simulink model "sixdof"  (R2022b)
settings: Solver=VariableStepAuto  StartTime=0.0  StopTime=10  RelTol=1e-3
undefined symbols (not defined in the file or in its folder): sigbuilder_block
libraries: matrix_library x1, shared6dof x1
settings Model: Creator=Freddie  LastModifiedBy=Freddie

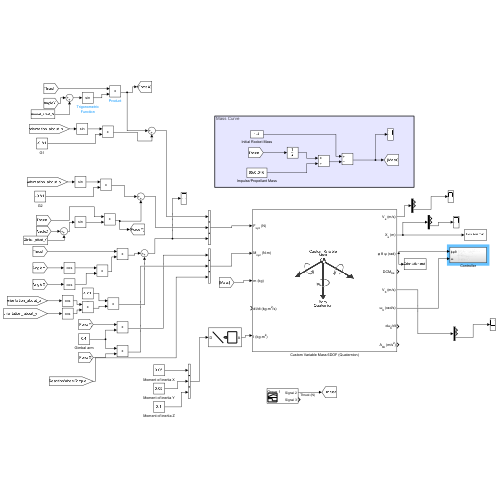
[thumbnail: Simulink's stored preview of the top-level diagram]
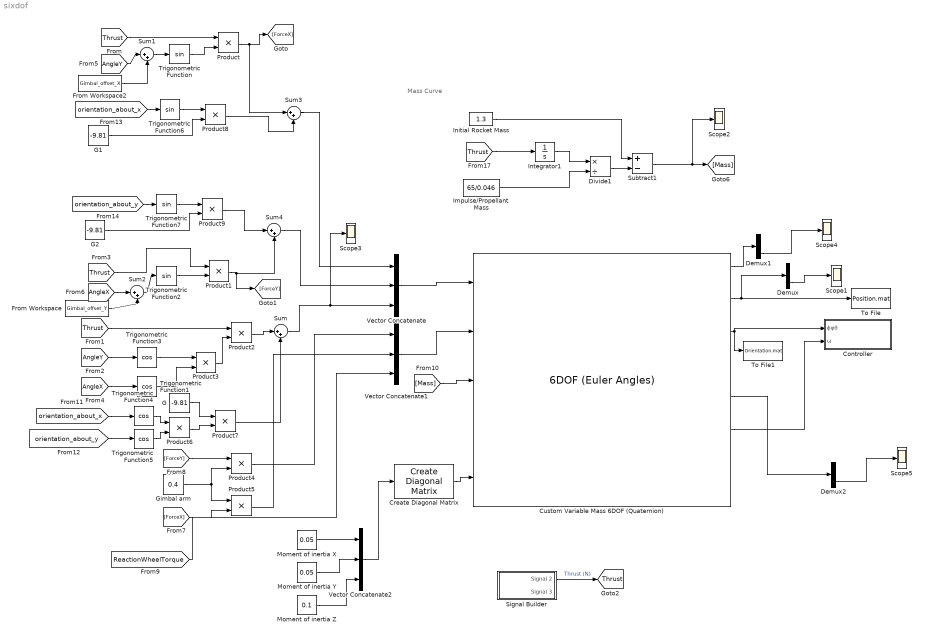
== system sixdof ==
  note: Mass Curve
  Controller : Subsystem
  Create Diagonal Matrix : matrix_library/Create Diagonal Matrix
      settings: LibrarySourceBlock=|
      | simulink/Matrix
      | Operations/Create Diagonal
      | Matrix
  Custom Variable Mass 6DOF (Quaternion) : shared6dof/6DOF (Euler Angles)  units=Metric (MKS)  mtype=Custom Variable  rep=Quaternion  xme_0=[0 0 0]  Vm_0=[0 0 0]  eul_0="[0 0 0  ]"  pm_0=[0 0 0]  mass_0=1.0  mass_e=0.5  mass_f=2.0  inertia=eye(3)  inertia_e=eye(3)  inertia_f=2*eye(3)  k_quat=1.0  vre_flag=off  abi_flag=off  aMode=0  xme_statename=''  Vm_statename=''  eul_statename=''  quat_statename=''  pm_statename=''  mass_statename=''
      settings: LibrarySourceBlock=aerolib6dof2/Custom Variable Mass 6DOF (Quaternion)
  Demux : Demux  Outputs=3
  Demux1 : Demux  Outputs=3
  Demux2 : Demux  Outputs=3
  Divide1 : Product  Inputs=*/
  From Workspace : FromWorkspace  VariableName=Gimbal_offset_Y  OutputAfterFinalValue=Holding final value
  From Workspace2 : FromWorkspace  VariableName=Gimbal_offset_X  OutputAfterFinalValue=Holding final value
  G : Constant  Value=-9.81
  G1 : Constant  Value=-9.81
  G2 : Constant  Value=-9.81
  Gimbal arm : Constant  Value=0.4
  Impulse/Propellant Mass : Constant  Value=65/0.046
  Initial Rocket Mass : Constant  Value=1.3
  Integrator1 : Integrator
  Moment of inertia X : Constant  Value=0.05
  Moment of inertia Y : Constant  Value=0.05
  Moment of inertia Z : Constant  Value=0.1
  Product{,1..9} (10 alike) : Product
  Scope{1..5} (5 alike) : Scope
  Signal Builder : Subsystem  Tag=STV Subsys  LoadFcn=sigbuilder_block('load');  StartFcn=sigbuilder_block('start');  StopFcn=sigbuilder_block('stop');  ClipboardFcn=sigbuilder_block('clipboard');  mask(Sigbuilder block){tuvar=[0:10]}
      mask help: Simulink:masks:SigbuilderBlock_MD
      mask init:
      | if ~strcmp(get_param(bdroot(gcbh),'SimulationStatus'),'stopped') tuvar = sigbuilder_block('maskInit'); end
      settings: CopyFcn=sigbuilder_block('copy');  DeleteFcn=sigbuilder_block('delete');  ModelCloseFcn=sigbuilder_block('modelClose');  PreSaveFcn=sigbuilder_block('preSave');  PauseFcn=sigbuilder_block('pause');  ContinueFcn=sigbuilder_block('continue');  NameChangeFcn=sigbuilder_block('namechange');  OpenFcn=sigbuilder_block('open',[437.6 199.2 550.4 400 ]);  CloseFcn=sigbuilder_block('close');
      mask Display: plot(0, 0, 100, 100,[2, 2, 32, 32, 2], [68, 8, 8, 68, 68],[32, 2], [38, 38], [32, 19, 2],[53, 60, 44], [32, 17, 17, 2],[16, 16, 31, 31]);txt = getActiveGroup(gcbh);text(2, 100, txt,'verticalAlignment', 'top');
  Subtract1 : Sum  Inputs=+-
  Sum{,1..4} (5 alike) : Sum  Inputs=|++
  To File : ToFile  Filename=Position.mat  MatrixName=Position  SampleTime=0.05
  To File1 : ToFile  Filename=Orientation.mat  MatrixName=Orientation  SampleTime=0.05
  Trigonometric Function{,2,6..7} (4 alike) : Trigonometry
  Trigonometric Function{1,3..5} (4 alike) : Trigonometry  Operator=cos
  Vector Concatenate : Concatenate  NumInputs=3
  Vector Concatenate1 : Concatenate  NumInputs=3
  Vector Concatenate2 : Concatenate  NumInputs=3
  tag scope: Thrust=global
  wires:
  [Thrust] -> Product/1
  Trigonometric Function/1 -> Product/2
  [Thrust] -> Product1/1
  Trigonometric Function2/1 -> Product1/2
  Trigonometric Function3/1 -> Product3/1
  Trigonometric Function1/1 -> Product3/2
  [Thrust] -> Product2/1
  Product3/1 -> Product2/2
  Product/1 -> Sum3/1, [ForceX]
  Product1/1 -> Sum4/2, [ForceY]
  [AngleY] -> Trigonometric Function3/1
  [AngleX] -> Trigonometric Function1/1
  Vector Concatenate/1 -> Custom Variable Mass 6DOF (Quaternion)/1
  Vector Concatenate1/1 -> Custom Variable Mass 6DOF (Quaternion)/2
  [ForceY] -> Product4/1
  [ForceX] -> Product5/2
  Gimbal arm/1 -> Product4/2, Product5/1
  [ReactionWheelTorque] -> Vector Concatenate1/3
  Signal Builder/1(Signal 2) -> [Thrust]  "Thrust (N)"
  Product2/1 -> Sum/1
  [Thrust] -> Integrator1/1
  Integrator1/1 -> Divide1/1
  Subtract1/1 -> Scope2/1, [Mass]
  Initial Rocket Mass/1 -> Subtract1/1
  Divide1/1 -> Subtract1/2
  Impulse/Propellant Mass/1 -> Divide1/2
  [Mass] -> Custom Variable Mass 6DOF (Quaternion)/3
  Create Diagonal Matrix/1 -> Custom Variable Mass 6DOF (Quaternion)/5
  Vector Concatenate2/1 -> Create Diagonal Matrix/1
  Moment of inertia Z/1 -> Vector Concatenate2/3
  Sum/1 -> Vector Concatenate/3, Scope3/1
  [AngleY] -> Sum1/1
  Sum1/1 -> Trigonometric Function/1
  [AngleX] -> Sum2/1
  Sum2/1 -> Trigonometric Function2/1
  From Workspace/1 -> Sum2/2
  From Workspace2/1 -> Sum1/2
  Custom Variable Mass 6DOF (Quaternion)/2 -> Demux/1, To File/1
  Custom Variable Mass 6DOF (Quaternion)/3 -> Controller/1(ϕφθ), To File1/1
  Custom Variable Mass 6DOF (Quaternion)/6 -> Controller/2(ω)
  Moment of inertia X/1 -> Vector Concatenate2/1
  Moment of inertia Y/1 -> Vector Concatenate2/2
  Product4/1 -> Vector Concatenate1/1
  Product5/1 -> Vector Concatenate1/2
  Demux/3 -> Scope1/1
  Custom Variable Mass 6DOF (Quaternion)/1 -> Demux1/1
  Demux1/3 -> Scope4/1
  Demux2/3 -> Scope5/1
  [orientation_about_x] -> Trigonometric Function4/1
  [orientation_about_y] -> Trigonometric Function5/1
  Trigonometric Function4/1 -> Product6/1
  Trigonometric Function5/1 -> Product6/2
  Product6/1 -> Product7/2
  G/1 -> Product7/1
  Product7/1 -> Sum/2
  [orientation_about_x] -> Trigonometric Function6/1
  Trigonometric Function6/1 -> Product8/1
  G1/1 -> Product8/2
  Product8/1 -> Sum3/2
  Sum3/1 -> Vector Concatenate/1
  [orientation_about_y] -> Trigonometric Function7/1
  Trigonometric Function7/1 -> Product9/1
  G2/1 -> Product9/2
  Product9/1 -> Sum4/1
  Sum4/1 -> Vector Concatenate/2
  Custom Variable Mass 6DOF (Quaternion)/5 -> Demux2/1

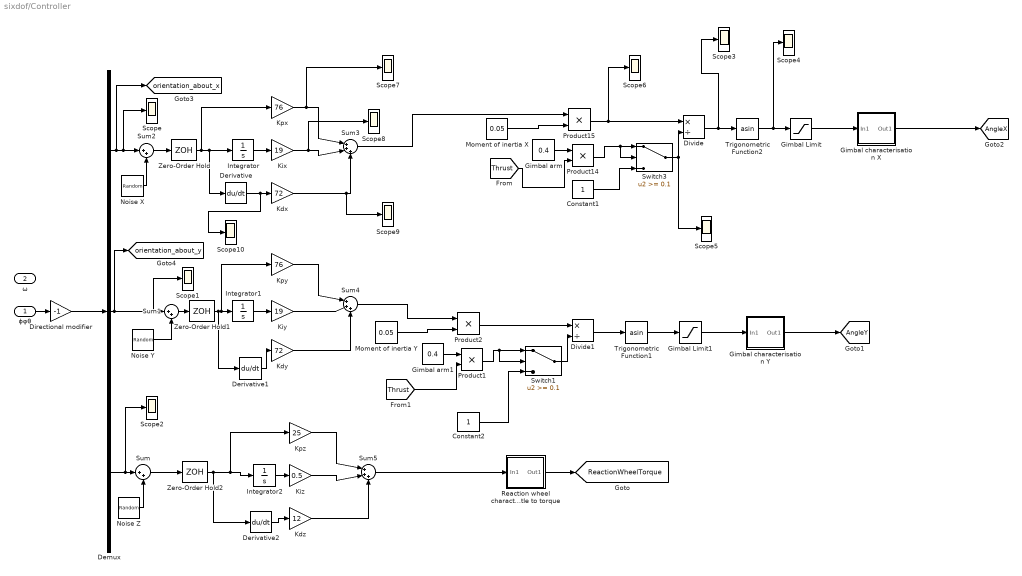
== system sixdof/Controller ==
  ϕφθ : Inport
  ω : Inport  Port=2
  Constant1 : Constant
  Constant2 : Constant
  Demux : Demux  Outputs=3
  Derivative : Derivative
  Derivative1 : Derivative
  Derivative2 : Derivative
  Directional modifier : Gain  Gain=-1
  Divide : Product  Inputs=*/
  Divide1 : Product  Inputs=*/
  Gimbal Limit : Saturate  UpperLimit=0.139626  LowerLimit=-0.139626
  Gimbal Limit1 : Saturate  UpperLimit=0.139626  LowerLimit=-0.139626
  Gimbal arm : Constant  Value=0.4
  Gimbal arm1 : Constant  Value=0.4
  Gimbal characterisation X : Subsystem
  Gimbal characterisation Y : Subsystem
  Integrator : Integrator
  Integrator1 : Integrator
  Integrator2 : Integrator
  Kdx : Gain  Gain=72
  Kdy : Gain  Gain=72
  Kdz : Gain  Gain=12
  Kix : Gain  Gain=19
  Kiy : Gain  Gain=19
  Kiz : Gain  Gain=0.5
  Kpx : Gain  Gain=76
  Kpy : Gain  Gain=76
  Kpz : Gain  Gain=25
  Moment of inertia X : Constant  Value=0.05
  Moment of inertia Y : Constant  Value=0.05
  Noise X : RandomNumber  Variance=0  SampleTime=0.1
  Noise Y : RandomNumber  Variance=0  SampleTime=0.1
  Noise Z : RandomNumber  Variance=0  Seed=2  SampleTime=0.1
  Product{1..2,14..15} (4 alike) : Product
  Reaction wheel characterization throttle to torque : Subsystem
  Scope{,1..10} (11 alike) : Scope
  Sum : Sum  Inputs=|++
  Sum1 : Sum  Inputs=|++
  Sum2 : Sum  Inputs=|++
  Sum3 : Sum  Inputs=|+++
  Sum4 : Sum  Inputs=|+++
  Sum5 : Sum  Inputs=|+++
  Switch1 : Switch  Threshold=0.1  SaturateOnIntegerOverflow=off  InputSameDT=off
  Switch3 : Switch  Threshold=0.1  SaturateOnIntegerOverflow=off  InputSameDT=off
  Trigonometric Function1 : Trigonometry  Operator=asin  OutputSignalType=real
  Trigonometric Function2 : Trigonometry  Operator=asin  OutputSignalType=real
  Zero-Order Hold : ZeroOrderHold  SampleTime=0.01
  Zero-Order Hold1 : ZeroOrderHold  SampleTime=0.01
  Zero-Order Hold2 : ZeroOrderHold  SampleTime=0.01
  tag scope: AngleX=global, AngleY=global, ReactionWheelTorque=global, orientation_about_x=global, orientation_about_y=global
  wires:
  Demux/3 -> Scope2/1, Sum/1
  Demux/1 -> [orientation_about_x], Scope/1, Sum2/1
  Demux/2 -> Scope1/1, Sum1/1, [orientation_about_y]
  Noise X/1 -> Sum2/2
  Noise Y/1 -> Sum1/2
  Noise Z/1 -> Sum/2
  Divide/1 -> Scope3/1, Trigonometric Function2/1
  Gimbal Limit/1 -> Gimbal characterisation X/1(In1)
  Product15/1 -> Scope6/1, Divide/1
  Trigonometric Function2/1 -> Scope4/1, Gimbal Limit/1
  Moment of inertia X/1 -> Product15/2
  Constant1/1 -> Switch3/3
  Gimbal arm/1 -> Product14/1
  Product14/1 -> Switch3/2, Switch3/1
  Switch3/1 -> Divide/2, Scope5/1
  Gimbal arm1/1 -> Product1/1
  Divide1/1 -> Trigonometric Function1/1
  Product2/1 -> Divide1/1
  Gimbal Limit1/1 -> Gimbal characterisation Y/1(In1)
  Trigonometric Function1/1 -> Gimbal Limit1/1
  Switch1/1 -> Divide1/2
  Constant2/1 -> Switch1/3
  Moment of inertia Y/1 -> Product2/2
  Reaction wheel characterization throttle to torque/1(Out1) -> [ReactionWheelTorque]
  Gimbal characterisation Y/1(Out1) -> [AngleY]
  Gimbal characterisation X/1(Out1) -> [AngleX]
  [Thrust] -> Product14/2
  [Thrust] -> Product1/2
  Product1/1 -> Switch1/2, Switch1/1
  Kpx/1 -> Scope7/1, Sum3/1
  Kix/1 -> Scope8/1, Sum3/2
  Kdx/1 -> Scope9/1, Sum3/3
  Kiy/1 -> Sum4/2
  Kpy/1 -> Sum4/1
  Kdy/1 -> Sum4/3
  Kiz/1 -> Sum5/2
  Kdz/1 -> Sum5/3
  Kpz/1 -> Sum5/1
  Sum5/1 -> Reaction wheel characterization throttle to torque/1(In1)
  Sum4/1 -> Product2/1
  Sum3/1 -> Product15/1
  Sum2/1 -> Zero-Order Hold/1
  Zero-Order Hold/1 -> Kpx/1, Derivative/1, Integrator/1
  Sum1/1 -> Zero-Order Hold1/1
  Zero-Order Hold1/1 -> Derivative1/1, Kpy/1, Integrator1/1
  Sum/1 -> Zero-Order Hold2/1
  Zero-Order Hold2/1 -> Derivative2/1, Kpz/1, Integrator2/1
  Integrator/1 -> Kix/1
  Integrator1/1 -> Kiy/1
  Integrator2/1 -> Kiz/1
  ϕφθ/1 -> Directional modifier/1
  Directional modifier/1 -> Demux/1
  Derivative1/1 -> Kdy/1
  Derivative2/1 -> Kdz/1
  Derivative/1 -> Scope10/1, Kdx/1

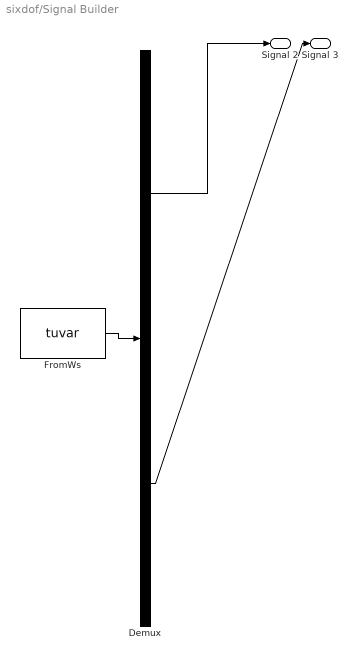
== system sixdof/Signal Builder ==
  Demux : Demux  Tag=STV Demux  Outputs=2
      settings: DisplayOption=none
  FromWs : FromWorkspace  Tag=STV FromWs  VariableName=tuvar
      SigBuilderData=|
      | common.afterFinalStr = 'Extrapolate'
      | common.sampleTime = 0
      | dataSet.timeRange = [0 10]
      | dataSet.name = 'Group 1'
      | sbobj.Groups.Name = 'Group 1'
      | sbobj.Groups.Signals(1).Name = 'Signal 2'
      | sbobj.Groups.Signals(1).XData = [0 0.014 0.075 0.157 0.293 0.382 0.45 0.539 0.614 0.662 0.771 0.948 0.996 1.078 1.187 1.289 1.337 1.412 1.474 1.515 1.542 1.706 1.938 2.101 2.129 2.251 2.402 2.64 2.961 3.31 10]
      | sbobj.Groups.Signals(1).YData = [11.527 11.527 20.126 26.572 29.113 30.278 29.69 30.667 30.089 31.15 30.478 29.89 28.714 28.136 27.738 26.761 26.96 25.984 25.008 26.173 24.808 22.856 20.903 18.173 19.338 16.21 13.48 8.791 3.32 0 0]
      | sbobj.Groups.Signals(2).Name = 'Signal 3'
      | sbobj.Groups.Signals(2).XData = [0 3.31 10]
      | sbobj.Groups.Signals(2).YData = [1.3 1.254 1.254]
  Signal 2 : Outport  Tag=STV Outport
  Signal 3 : Outport  Tag=STV Outport  Port=2
  wires:
  FromWs/1 -> Demux/1
  Demux/1 -> Signal 2/1
  Demux/2 -> Signal 3/1

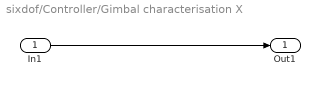
== system sixdof/Controller/Gimbal characterisation X ==
  In1 : Inport
  Out1 : Outport
  wires:
  In1/1 -> Out1/1

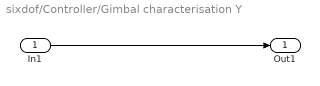
== system sixdof/Controller/Gimbal characterisation Y ==
  In1 : Inport
  Out1 : Outport
  wires:
  In1/1 -> Out1/1

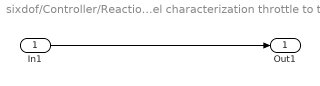
== system sixdof/Controller/Reaction wheel characterization throttle to torque ==
  In1 : Inport
  Out1 : Outport
  wires:
  In1/1 -> Out1/1
